simulink model "Simulink1"  (R2016a)
settings: Solver=VariableStepAuto  StartTime=0.0  StopTime=1  MinStep=0.001  RelTol=1e-3
values from neighbouring files (symbols this model uses):
  C = [-1 0 1 0]    [Data.m]
  Cac = A(4,:)    [Data.m]
  Dac = 1/M2    (= 0.004)    [Data.m]
  K = lqr(A,B,Qx,R,N)    [Data.m]
  M2 = 250    [Data.m]
  X0 = [0.0022, -0.1146, 0.0421, -0.0138]'    [Data.m]
libraries: commchan3 x5
settings Model: Creator=NAD  LastModifiedBy=NAD

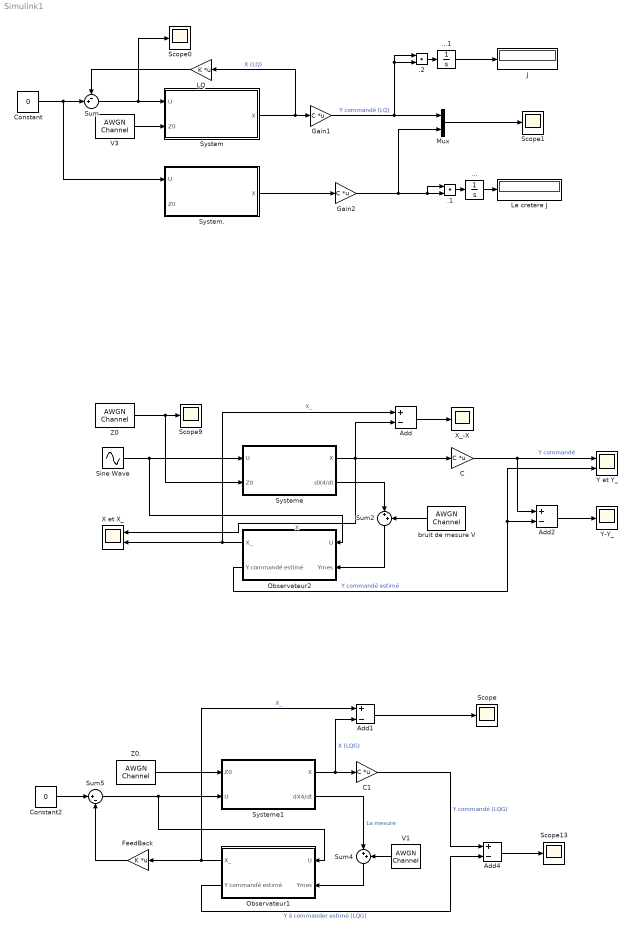
== system Simulink1 ==
  ... : Integrator
  ...1 : Integrator
  .1 : DotProduct  InputSameDT=on  OutDataTypeStr=Inherit: Inherit via internal rule
  .2 : DotProduct  InputSameDT=on  OutDataTypeStr=Inherit: Inherit via internal rule
  Add{,1..2,4} (4 alike) : Sum  Inputs=+-
  C : Gain  Gain=C  Multiplication=Matrix(K*u) (u vector)
  C1 : Gain  Gain=C  Multiplication=Matrix(K*u) (u vector)
  Constant : Constant  Value=0
  Constant2 : Constant  Value=0
  FeedBack : Gain  Gain=K  Multiplication=Matrix(K*u) (u vector)
  Gain1 : Gain  Gain=C  Multiplication=Matrix(K*u) (u vector)
  Gain2 : Gain  Gain=C  Multiplication=Matrix(K*u) (u vector)
  J : Display
  LQ : Gain  Gain=K  Multiplication=Matrix(K*u) (u vector)
  Le cretere J : Display
  Mux : Mux  Inputs=2
  Observateur1 : Subsystem
  Observateur2 : Subsystem
  Scope{,0..1,9,13} (5 alike) : Scope
  Sine Wave : Sin  SampleTime=0
  Sum : Sum  Inputs=-+|
  Sum2 : Sum  Inputs=|++
  Sum4 : Sum  Inputs=|++
  Sum5 : Sum  Inputs=|+-
  System : Subsystem
  System. : Subsystem
  Systeme : Subsystem
  Systeme1 : Subsystem
  V1 : commchan3/AWGN Channel  InputProcessing=Columns as channels (frame based)  seed=67  noiseMode=Variance from mask  EbNodB=10  EsNodB=10  SNRdB=10  bitsPerSym=1  Ps=1  Tsym=1  variance=r1
  V3 : commchan3/AWGN Channel  InputProcessing=Columns as channels (frame based)  seed=67  noiseMode=Variance from mask  EbNodB=10  EsNodB=10  SNRdB=10  bitsPerSym=1  Ps=1  Tsym=1  variance=0.01
  X et X_ : Scope  NumInputPorts=2
  X_-X : Scope
  Y et Y_ : Scope  NumInputPorts=2
  Y-Y_ : Scope
  Z0 : commchan3/AWGN Channel  InputProcessing=Inherited (this choice will be removed - see release notes)  seed=67  noiseMode=Variance from mask  EbNodB=10  EsNodB=10  SNRdB=10  bitsPerSym=1  Ps=1  Tsym=1  variance=0.01
  Z0. : commchan3/AWGN Channel  InputProcessing=Columns as channels (frame based)  seed=67  noiseMode=Variance from mask  EbNodB=10  EsNodB=10  SNRdB=10  bitsPerSym=1  Ps=1  Tsym=1  variance=r0
  bruit de mesure V : commchan3/AWGN Channel  InputProcessing=Columns as channels (frame based)  seed=67  noiseMode=Variance from mask  EbNodB=10  EsNodB=10  SNRdB=10  bitsPerSym=1  Ps=1  Tsym=1  variance=0.01
  wires:
  System/1(X) -> Gain1/1, LQ/1  "X (LQ)"
  LQ/1 -> Sum/1
  Constant/1 -> System./1(U), Sum/2
  Sum/1 -> Scope0/1, System/1(U)
  Mux/1 -> Scope1/1
  System./1(X) -> Gain2/1
  Gain2/1 -> .1/1, .1/2, Mux/2
  Sine Wave/1 -> Observateur2/1(U), Systeme/1(U)
  C/1 -> Y et Y_/1, Add2/1  "Y commandé"
  Systeme/1(X) -> Add/2, X et X_/1, C/1  "X"
  Observateur2/1(X_) -> X et X_/2, Add/1  "X_"
  Systeme/2(dX4/dt) -> Sum2/1
  Z0/1 -> Systeme/2(Z0), Scope9/1
  bruit de mesure V/1 -> Sum2/2
  Sum2/1 -> Observateur2/2(Ymes)
  Sum5/1 -> Systeme1/2(U), Observateur1/1(U)
  C1/1 -> Add4/1  "Y commandé (LQG)"
  Systeme1/2(dX4/dt) -> Sum4/1  "La mesure"
  Constant2/1 -> Sum5/1
  Sum4/1 -> Observateur1/2(Ymes)
  Systeme1/1(X) -> Add1/2, C1/1  "X (LQG)"
  FeedBack/1 -> Sum5/2
  .1/1 -> .../1
  .../1 -> Le cretere J/1
  ...1/1 -> J/1
  Observateur1/1(X_) -> Add1/1, FeedBack/1  "X_"
  Gain1/1 -> Mux/1, .2/2, .2/1  "Y commandé (LQ)"
  .2/1 -> ...1/1
  Add2/1 -> Y-Y_/1
  V1/1 -> Sum4/2
  Observateur1/2("Y commandé estimé ") -> Add4/2  "Y á commander estimé (LQG)"
  Add1/1 -> Scope/1
  Add4/1 -> Scope13/1
  Z0./1 -> Systeme1/1(Z0)
  Add/1 -> X_-X/1
  V3/1 -> System/2(Z0)
  Observateur2/2("Y commandé estimé ") -> Y et Y_/2, Add2/2  "Y commandé estimé"

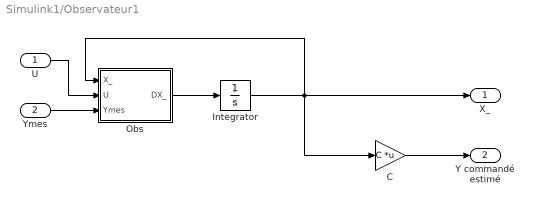
== system Simulink1/Observateur1 ==
  U : Inport
  Ymes : Inport  Port=2
  C : Gain  Gain=C  Multiplication=Matrix(K*u) (u vector)
  Integrator : Integrator  InitialCondition=[0.3 1 0.9 1]'*0+X0
  Obs : MATLAB Function  TreatAsAtomicUnit=on
  X_ : Outport
  "Y commandé estimé " : Outport  Port=2
  wires:
  U/1 -> Obs/2(U)
  Integrator/1 -> C/1, Obs/1(X_), X_/1
  Obs/1(DX_) -> Integrator/1
  Ymes/1 -> Obs/3(Ymes)
  C/1 -> "Y commandé estimé "/1

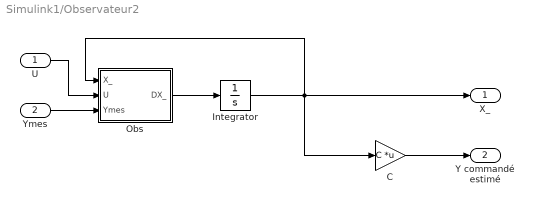
== system Simulink1/Observateur2 ==
  U : Inport
  Ymes : Inport  Port=2
  C : Gain  Gain=C  Multiplication=Matrix(K*u) (u vector)
  Integrator : Integrator  InitialCondition=[0.3 1 0.9 1]'+X0
  Obs : MATLAB Function  TreatAsAtomicUnit=on
  X_ : Outport
  "Y commandé estimé " : Outport  Port=2
  wires:
  U/1 -> Obs/2(U)
  Integrator/1 -> C/1, Obs/1(X_), X_/1
  Obs/1(DX_) -> Integrator/1
  Ymes/1 -> Obs/3(Ymes)
  C/1 -> "Y commandé estimé "/1

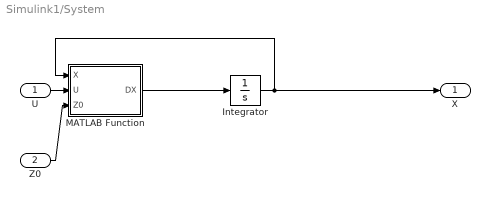
== system Simulink1/System ==
  U : Inport
  Z0 : Inport  Port=2
  Integrator : Integrator  InitialCondition=[0.0022, -0.1146, 0.0421, -0.0138]'
  MATLAB Function : MATLAB Function  TreatAsAtomicUnit=on
  X : Outport
  wires:
  MATLAB Function/1(DX) -> Integrator/1
  Integrator/1 -> X/1, MATLAB Function/1(X)
  Z0/1 -> MATLAB Function/3(Z0)
  U/1 -> MATLAB Function/2(U)

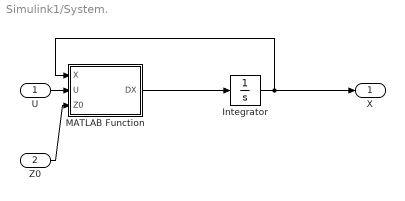
== system Simulink1/System. ==
  U : Inport
  Z0 : Inport  Port=2
  Integrator : Integrator  InitialCondition=[0.0022, -0.1146, 0.0421, -0.0138]'
  MATLAB Function : MATLAB Function  TreatAsAtomicUnit=on
  X : Outport
  wires:
  U/1 -> MATLAB Function/2(U)
  Z0/1 -> MATLAB Function/3(Z0)
  Integrator/1 -> MATLAB Function/1(X), X/1
  MATLAB Function/1(DX) -> Integrator/1

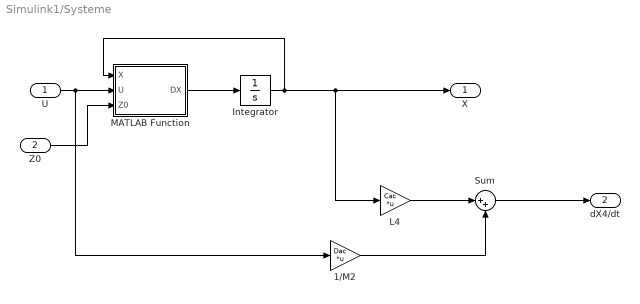
== system Simulink1/Systeme ==
  U : Inport
  Z0 : Inport  Port=2
  1/M2 : Gain  Gain=Dac  Multiplication=Matrix(K*u) (u vector)
  Integrator : Integrator  InitialCondition=X0
  "L4 " : Gain  Gain=Cac  Multiplication=Matrix(K*u) (u vector)
  MATLAB Function : MATLAB Function  TreatAsAtomicUnit=on
  Sum : Sum  Inputs=|++
  X : Outport
  dX4/dt : Outport  Port=2
  wires:
  MATLAB Function/1(DX) -> Integrator/1
  Integrator/1 -> "L4 "/1, X/1, MATLAB Function/1(X)
  Z0/1 -> MATLAB Function/3(Z0)
  U/1 -> MATLAB Function/2(U), 1/M2/1
  "L4 "/1 -> Sum/1
  Sum/1 -> dX4/dt/1
  1/M2/1 -> Sum/2

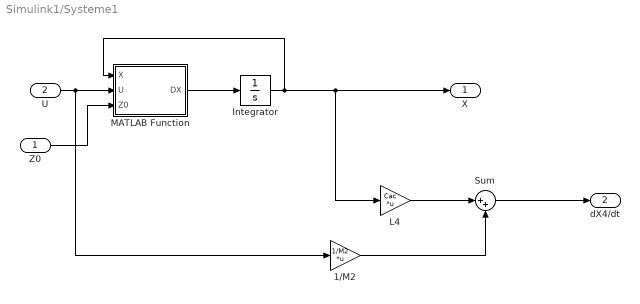
== system Simulink1/Systeme1 ==
  Z0 : Inport
  U : Inport  Port=2
  1/M2 : Gain  Gain=1/M2  Multiplication=Matrix(K*u) (u vector)
  Integrator : Integrator  InitialCondition=[0.0022, -0.1146, 0.0421, -0.0138]'
  "L4 " : Gain  Gain=Cac  Multiplication=Matrix(K*u) (u vector)
  MATLAB Function : MATLAB Function  TreatAsAtomicUnit=on
  Sum : Sum  Inputs=|++
  X : Outport
  dX4/dt : Outport  Port=2
  wires:
  MATLAB Function/1(DX) -> Integrator/1
  Integrator/1 -> "L4 "/1, X/1, MATLAB Function/1(X)
  Z0/1 -> MATLAB Function/3(Z0)
  U/1 -> MATLAB Function/2(U), 1/M2/1
  "L4 "/1 -> Sum/1
  Sum/1 -> dX4/dt/1
  1/M2/1 -> Sum/2

== matlab function Simulink1/System./MATLAB Function ==
  data: X input; DX output; U input; Z0 input
function DX = fcn(X,U,Z0)

M1 = 30; M2 = 250; k= 2*10^4; k1 = 2*10^5; f = 1000;
A = [ 0 1 0 0
      -(k1+k)/M1 -f/M1 k/M1 f/M1
      0            0    0     1
      k/M2        f/M2   -k/M2  -f/M2];
B = [0; -1/M1; 0; 1/M2];
Bp = [0; k1/M1; 0 ; 0];


DX = A*X+B*U+Bp*Z0;
end

== matlab function Simulink1/System/MATLAB Function ==
  data: X input; DX output; U input; Z0 input
function DX = fcn(X,U,Z0)

M1 = 30; M2 = 250; k= 2*10^4; k1 = 2*10^5; f = 1000;
A = [ 0 1 0 0
      -(k1+k)/M1 -f/M1 k/M1 f/M1
      0            0    0     1
      k/M2        f/M2   -k/M2  -f/M2];
B = [0; -1/M1; 0; 1/M2];
Bp = [0; k1/M1; 0 ; 0];


DX = A*X+B*U+Bp*Z0;
end

== matlab function Simulink1/Systeme/MATLAB Function ==
  data: X input; DX output; U input; Z0 input
function DX = fcn(X,U,Z0)

M1 = 30; M2 = 250; k= 2*10^4; k1 = 2*10^5; f = 1000;
A = [ 0 1 0 0
      -(k1+k)/M1 -f/M1 k/M1 f/M1
      0            0    0     1
      k/M2        f/M2   -k/M2  -f/M2];
B = [0; -1/M1; 0; 1/M2];
Bp = [0; k1/M1; 0 ; 0];


DX = A*X + B*U + Bp*Z0 ;
end

== matlab function Simulink1/Observateur2/Obs ==
  data: X_ input; DX_ output; U input; Ymes input
function DX_ = fcn(X_,U,Ymes)

M1 = 30; M2 = 250; k= 2*10^4; k1 = 2*10^5; f = 1000;
A = [ 0 1 0 0
      -(k1+k)/M1 -f/M1 k/M1 f/M1
      0            0    0     1
      k/M2        f/M2   -k/M2  -f/M2];
B = [0; -1/M1; 0; 1/M2];
C = A(4,:);
D = 1/M2;
% r0 = 0.01
Kf =1.0e+03 *[

   -0.0012
    6.6577
   -0.0014
   -0.00000] ;
% r0=1
Kf = 1.0e+04 *[

   -0.0004
    6.6657
   -0.0004
   -0.0000];

Ymes_ = C*X_ + D*U ;
DX_ = A*X_ + B*U + Kf*(Ymes - Ymes_);

end

== matlab function Simulink1/Observateur1/Obs ==
  data: X_ input; DX_ output; U input; Ymes input
function DX_ = fcn(X_,U,Ymes)

M1 = 30; M2 = 250; k= 2*10^4; k1 = 2*10^5; f = 1000;
A = [ 0 1 0 0
      -(k1+k)/M1 -f/M1 k/M1 f/M1
      0            0    0     1
      k/M2        f/M2   -k/M2  -f/M2];
B = [0; -1/M1; 0; 1/M2];
C = A(4,:);
D = 1/M2;
Kf =1.0e+03 *[

   -0.0012
    6.6577
   -0.0014
   -0.00000] ;

Ymes_ = C*X_ + D*U ;
DX_ = A*X_ + B*U + Kf*(Ymes - Ymes_);

end

== matlab function Simulink1/Systeme1/MATLAB Function ==
  data: X input; DX output; U input; Z0 input
function DX = fcn(X,U,Z0)

M1 = 30; M2 = 250; k= 2*10^4; k1 = 2*10^5; f = 1000;
A = [ 0 1 0 0
      -(k1+k)/M1 -f/M1 k/M1 f/M1
      0            0    0     1
      k/M2        f/M2   -k/M2  -f/M2];
B = [0; -1/M1; 0; 1/M2];
Bp = [0; k1/M1; 0 ; 0];


DX = A*X + B*U + Bp*Z0 ;
end
